simulink model "lab1_model3"  (R2021b)
settings: Solver=VariableStepAuto  StartTime=0.0  StopTime=60  RelTol=1e-3
undefined symbols (not defined in the file or in its folder): K_B
libraries: cstblocks x6
settings Model: Creator=12288  LastModifiedBy=12288

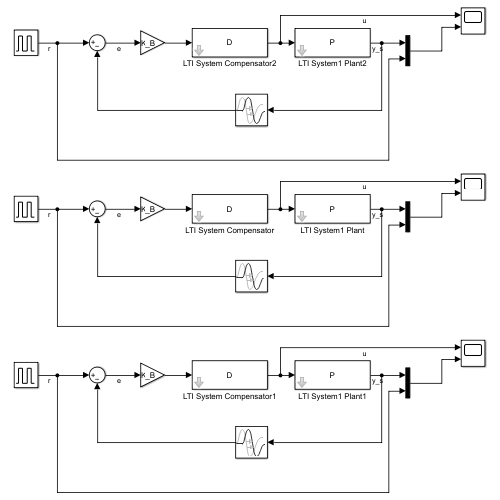
[thumbnail: Simulink's stored preview of the top-level diagram]
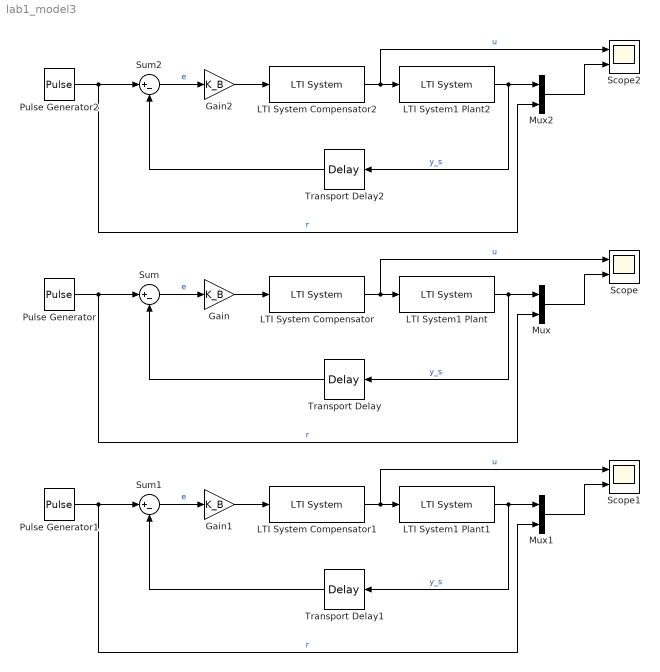
== system lab1_model3 ==
  Gain : Gain  Gain=K_B
  Gain1 : Gain  Gain=K_B
  Gain2 : Gain  Gain=K_B
  LTI System Compensator : cstblocks/LTI System  sys=D  IC=[]
  LTI System Compensator1 : cstblocks/LTI System  sys=D  IC=[]
  LTI System Compensator2 : cstblocks/LTI System  sys=D  IC=[]
  LTI System1 Plant : cstblocks/LTI System  sys=P  IC=[]
  LTI System1 Plant1 : cstblocks/LTI System  sys=P  IC=[]
  LTI System1 Plant2 : cstblocks/LTI System  sys=P  IC=[]
  Mux : Mux  Inputs=2
  Mux1 : Mux  Inputs=2
  Mux2 : Mux  Inputs=2
  Pulse Generator : DiscretePulseGenerator  PulseType=Time based  Period=10  PulseWidth=5
  Pulse Generator1 : DiscretePulseGenerator  PulseType=Time based  Period=10  PulseWidth=5
  Pulse Generator2 : DiscretePulseGenerator  PulseType=Time based  Period=10  PulseWidth=5
  Scope : Scope  NumInputPorts=2
  Scope1 : Scope  NumInputPorts=2
  Scope2 : Scope  NumInputPorts=2
  Sum : Sum  Inputs=|+-
  Sum1 : Sum  Inputs=|+-
  Sum2 : Sum  Inputs=|+-
  Transport Delay : TransportDelay  DelayTime=0.02
  Transport Delay1 : TransportDelay  DelayTime=0.03
  Transport Delay2 : TransportDelay  DelayTime=0.023
  wires:
  Mux/1 -> Scope/2
  LTI System Compensator/1 -> Scope/1, LTI System1 Plant/1  "u"
  Gain/1 -> LTI System Compensator/1
  LTI System1 Plant/1 -> Transport Delay/1, Mux/1  "y_s"
  Sum/1 -> Gain/1  "e"
  Pulse Generator/1 -> Mux/2, Sum/1  "r"
  Transport Delay/1 -> Sum/2
  Sum1/1 -> Gain1/1  "e"
  LTI System1 Plant1/1 -> Transport Delay1/1, Mux1/1  "y_s"
  Transport Delay1/1 -> Sum1/2
  Pulse Generator1/1 -> Mux1/2, Sum1/1  "r"
  Gain1/1 -> LTI System Compensator1/1
  LTI System Compensator1/1 -> Scope1/1, LTI System1 Plant1/1  "u"
  Mux1/1 -> Scope1/2
  Mux2/1 -> Scope2/2
  LTI System1 Plant2/1 -> Transport Delay2/1, Mux2/1  "y_s"
  Transport Delay2/1 -> Sum2/2
  Gain2/1 -> LTI System Compensator2/1
  LTI System Compensator2/1 -> Scope2/1, LTI System1 Plant2/1  "u"
  Pulse Generator2/1 -> Mux2/2, Sum2/1  "r"
  Sum2/1 -> Gain2/1  "e"
